simulink model "mylab2_simulink_to_ros"  (R2017a)
settings: Solver=FixedStepAuto  StartTime=0.0  StopTime=10.0  FixedStep=0.1  RelTol=1e-3
undefined symbols (not defined in the file): Rpm1, Rpm2, Rpm3, Rpm4
libraries: robotlib x7
settings Model: Creator=edward  LastModifiedBy=root
settings OptimizationCC: PassReuseOutputArgsAs=Individual arguments  MaxStackSize=64
settings DebuggingCC: ParameterTunabilityLossMsg=error
settings HardwareCC: ProdBitPerLong=64  ProdHWDeviceType=Intel->x86-64 (Linux 64)
settings SFSimCC: MATLABDynamicMemAlloc=off
settings RTWCC: SystemTargetFile=ert.tlc  HardwareBoard=Robot Operating System (ROS)  TLCOptions="-aInlineSetEventsForThisBaseRateFcn=TLC_FALSE -aSuppressMultiTaskScheduler=TLC_FALSE  -aRateBasedStepFcn=0"  TemplateMakefile=ert_default_tmf  Description=Embedded Coder  GenerateReport=on  Toolchain=Catkin  IncludeHyperlinkInReport=on  LaunchReport=on  TargetLang=C++  GenerateTraceInfo=on  GenerateTraceReport=on  GenerateTraceReportSl=on  GenerateTraceReportSf=on  GenerateTraceReportEml=on
settings CodeAppCC: ForceParamTrailComments=on  IgnoreCustomStorageClasses=off  OperatorAnnotations=on  SimulinkDataObjDesc=on  SFDataObjDesc=on  MATLABFcnDesc=on  InsertBlockDesc=on  MATLABSourceComments=on
settings ERTTargetCC: SupportContinuousTime=on

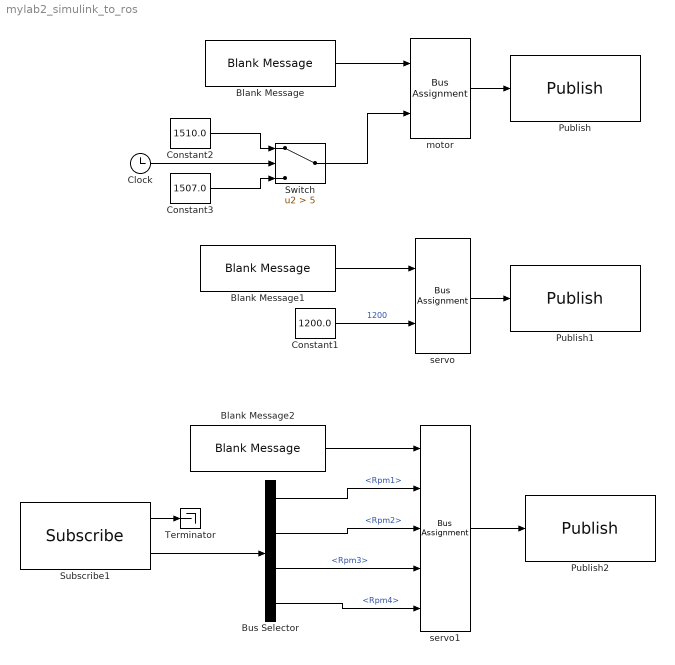
== system mylab2_simulink_to_ros ==
  Blank Message : robotlib/Blank Message  SourceLibraryInfo=This block requires Robotics System Toolbox  messageType=std_msgs/Float32  SampleTime=inf
      settings: SourceProductBaseCode=RO
  Blank Message1 : robotlib/Blank Message  SourceLibraryInfo=This block requires Robotics System Toolbox  messageType=std_msgs/Float32  SampleTime=inf
      settings: SourceProductBaseCode=RO
  Blank Message2 : robotlib/Blank Message  SourceLibraryInfo=This block requires Robotics System Toolbox  messageType=arduino_sub_pub/msgs_type  SampleTime=inf
      settings: SourceProductBaseCode=RO
  Bus Selector : BusSelector  OutputSignals=Rpm1,Rpm2,Rpm3,Rpm4
  Clock : Clock
      settings: Decimation=1000
  Constant1 : Constant  Value=1200.0  OutDataTypeStr=single
  Constant2 : Constant  Value=1510.0  OutDataTypeStr=single
  Constant3 : Constant  Value=1507.0  OutDataTypeStr=single
  Publish : robotlib/Publish  SourceLibraryInfo=This block requires Robotics System Toolbox  topicSource=Specify your own  topic=/motor_pwm  messageType=std_msgs/Float32  messageQueueLength=1
      settings: SourceProductBaseCode=RO
  Publish1 : robotlib/Publish  SourceLibraryInfo=This block requires Robotics System Toolbox  topicSource=Specify your own  topic=/servo_pwm  messageType=std_msgs/Float32  messageQueueLength=1
      settings: SourceProductBaseCode=RO
  Publish2 : robotlib/Publish  SourceLibraryInfo=This block requires Robotics System Toolbox  topicSource=Specify your own  topic=/hall_publisher_ed  messageType=arduino_sub_pub/msgs_type  messageQueueLength=1
      settings: SourceProductBaseCode=RO
  Subscribe1 : robotlib/Subscribe  SourceLibraryInfo=This block requires Robotics System Toolbox  topicSource=Specify your own  topic=/hall_parsing_data  messageType=arduino_sub_pub/msgs_type  sampleTime=-1  messageQueueLength=1
      settings: SourceProductBaseCode=RO
  Switch : Switch  Criteria=u2 > Threshold  Threshold=5
  Terminator : Terminator
  motor : BusAssignment  AssignedSignals=Data
  servo : BusAssignment  AssignedSignals=Data
  servo1 : BusAssignment  AssignedSignals=Rpm1,Rpm2,Rpm3,Rpm4
  wires:
  Blank Message/1 -> motor/1
  motor/1 -> Publish/1
  Constant1/1 -> servo/2  "1200"
  servo/1 -> Publish1/1
  Blank Message1/1 -> servo/1
  Constant2/1 -> Switch/1
  Clock/1 -> Switch/2
  Switch/1 -> motor/2
  Constant3/1 -> Switch/3
  Subscribe1/2 -> Bus Selector/1
  Subscribe1/1 -> Terminator/1
  Blank Message2/1 -> servo1/1
  Bus Selector/1 -> servo1/2  "<Rpm1>"
  Bus Selector/2 -> servo1/3  "<Rpm2>"
  Bus Selector/3 -> servo1/4  "<Rpm3>"
  Bus Selector/4 -> servo1/5  "<Rpm4>"
  servo1/1 -> Publish2/1
